simulink model "F16_Without_anti_HWP"  (R2022a)
settings: Solver=ode4  StartTime=0.0  StopTime=200  FixedStep=0.01  RelTol=1e-5  AbsTol=1e-4  EnableMultiTasking=on
InitFcn:
  | F16_Real5_init
libraries: etargetslib x10, dspnetwork x9, simulink x2, vrlib x1
settings Model: SimulationMode=accelerator  Creator=WhisPer  LastModifiedBy=lzj
settings SolverCC: AutoScaleAbsTol=off  AlgebraicLoopSolver=TrustRegion
settings DataIOCC: LimitDataPoints=on  SaveFormat=Array  ReturnWorkspaceOutputs=off
settings OptimizationCC: LifeSpan=inf
settings DebuggingCC: UnderspecifiedInitializationDetection=Classic  MergeDetectMultiDrivingBlocksExec=none  SolverPrmCheckMsg=warning  UnconnectedInputMsg=warning  UnconnectedOutputMsg=warning  UnconnectedLineMsg=warning  StateNameClashWarn=warning  SFUnexpectedBacktrackingDiag=warning  SFNoUnconditionalDefaultTransitionDiag=warning  SFExecutionAtInitializationDiag=none  SFMachineParentedDataDiag=warning  ArithmeticOperatorsInVariantConditions=warning
settings HardwareCC: ProdBitPerPointer=32  ProdBitPerSizeT=32  ProdBitPerPtrDiffT=32  ProdLargestAtomicFloat=None  ProdIntDivRoundTo=Undefined  ProdEndianess=Unspecified  ProdWordSize=32  ProdHWDeviceType=32-bit Generic
settings ModelReferenceCC: PropagateSignalLabelsOutOfModel=off
settings SFSimCC: SimUseLocalCustomCode=off  CustomCodeUndefinedFunction=UseInterfaceOnly
settings RTWCC: RTWUseLocalCustomCode=off
settings CodeAppCC: StateflowObjectComments=on
settings GRTTargetCC: TargetLangStandard=C89/C90 (ANSI)
settings ConfigComp: CovMetricSettings=dw  CovSaveCumulativeToWorkspaceVar=on  CovSaveSingleToWorkspaceVar=on  CovExternalEMLEnable=off

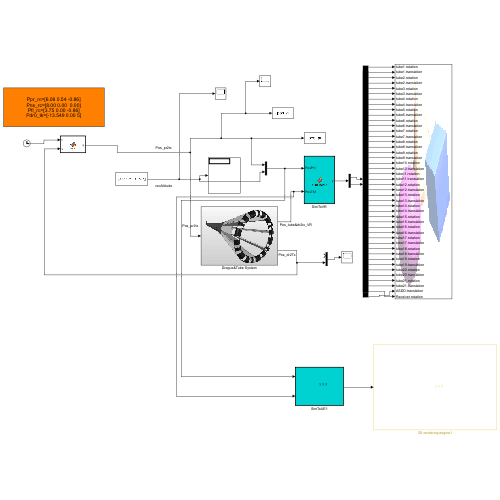
[thumbnail: Simulink's stored preview of the top-level diagram]
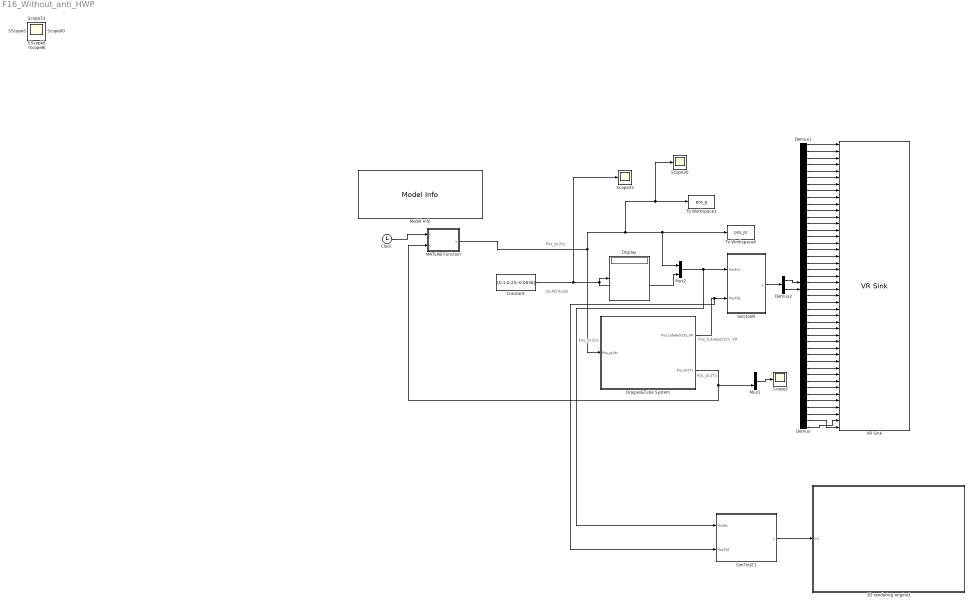
== system F16_Without_anti_HWP ==
  note: recAttitude
  note: Pos_dr2Tx
  note: Pos_tube&dr2tx_VR
  note: Pos_pr2tx
  note: Pos_pr2tx
  3D rendering engine1 : Subsystem
      mask Display: image('C:\Users\lgy13\Desktop\当下要完成的\AirRefueling3DVR-Blank\Icon\sideview.png'); % Use "Edit Image" on toolstrip to change.
  Clock : Clock
  Constant : Constant  Value=[0.1;0.25;-0.0636]
  Demux : Demux  Outputs=22
  Demux1 : Demux  Outputs=22
  Demux2 : Demux  Outputs=[88,66]
  Display : Display
  Drague&Tube System : Subsystem
      mask Display: image(imread('Icon\zhuitao.png'))
  MATLAB Function : MATLAB Function  TreatAsAtomicUnit=on
  Model Info : simulink/Model-Wide Utilities/Model Info  Frame=on  DisplayStringWithTags=|  HorizontalTextAlignment=Center  LeftAlignmentValue=0.5
      | Ppr_rc=[6.06 0.54 -0.86]
      | Pns_rc=[8.00 0.00  0.00]
      | Pfl_rc=[3.75 0.00 -0.86]
      | Pdr0_tk=[-13.549 0.00 5]
  Mux1 : Mux  Inputs=2
  Mux2 : Mux  Inputs=2
  Scope{,1..36} (37 alike) : Scope
  SimToUE1 : MATLAB Function  TreatAsAtomicUnit=on
  SimToVR : MATLAB Function  TreatAsAtomicUnit=on
  To Workspace3 : ToWorkspace  VariableName=pos_g  SampleTime=-1
  To Workspace4 : ToWorkspace  VariableName=pos_pr  SampleTime=-1
  VR Sink : vrlib/VR Sink  InstantiateOnLoad=on  SampleTime=-1  ViewEnable=on  RemoteChange=off  RemoteView=off  FieldsWritten=tube1.rotation.4.1.1.double#tube1.translation.3.1.1.double#tube2.rotation.4.1.1.double#tube2.translation.3.1.1.double#tube3.rotation.4.1.1.double#tube3.translation.3.1.1.double#tube4.rotation.4.1.1.double#tube4.translation.3.1.1.double#tube5.rotation.4.1.1.double#tube5.translation.3.1.1.double#tube6.rotation.4.1.1.double#tube6.translation.3.1.1.double#tube7.rotation.4.1.1.double#tube7.translation.3.1.1.double#tube8.rotation.4.1.1.double#tube8.translation.3.1.1.double#tube9.rotation.4.1.1.double#tube9.translation.3.1.1.double#tube10.rotation.4.1.1.double#tube10.translation.3.1.1.double#tube11.rotation.4.1.1.double#tube11.translation.3.1.1.double#tube12.rotation.4.1.1.double#tube12.translation.3.1.1.double#tube13.rotation.4.1.1.double#tube13.translation.3.1.1.double#tube14.rotation.4.1.1.double#tube14.translation.3.1.1.double#tube15.rotation.4.1.1.double#tube15.translation.3.1.1.double#tube16.rotation.4.1.1.double#tube16.translation.3.1.1.double#tube17.rotation.4.1.1.double#tube17.translation.3.1.1.double#tube18.rotation.4.1.1.double#tube18.translation.3.1.1.double#tube19.rotation.4.1.1.double#tube19.translation.3.1.1.double#tube20.rotation.4.1.1.double#tube20.translation.3.1.1.double#tube21.rotation.4.1.1.double#tube21.translation.3.1.1.double#ASDD.translation.3.1.1.double#Receiver.rotation.4.1.1.double  WorldFileName=AirRefuelingTubeSim.WRL  AutoView=off  VideoDimensions=[]  AllowVariableSize=off
  wires:
  MATLAB Function/1(y) -> Drague&Tube System/1(Pos_pr2tx), Mux2/1, To Workspace4/1, Scope36/1, To Workspace3/1
  Drague&Tube System/2(Pos_dr2Tx) -> MATLAB Function/2(v), Mux1/2
  Mux1/1 -> Scope2/1
  Constant/1 -> Scope35/1, Display/1, Mux2/2
  Demux2/2 -> Demux/1
  SimToVR/1(y) -> Demux2/1
  Drague&Tube System/1(Pos_tube&dr2tx_VR) -> SimToUE1/2(PosTb1), SimToVR/2(PosTb1)
  Mux2/1 -> SimToUE1/1(PosRc), SimToVR/1(PosPr1)
  Demux1/1 -> VR Sink/1
  Demux/1 -> VR Sink/2
  Demux1/2 -> VR Sink/3
  Demux/2 -> VR Sink/4
  Demux1/3 -> VR Sink/5
  Demux/3 -> VR Sink/6
  Demux1/4 -> VR Sink/7
  Demux/4 -> VR Sink/8
  Demux1/5 -> VR Sink/9
  Demux/5 -> VR Sink/10
  Demux1/6 -> VR Sink/11
  Demux/6 -> VR Sink/12
  Demux1/7 -> VR Sink/13
  Demux/7 -> VR Sink/14
  Demux1/8 -> VR Sink/15
  Demux/8 -> VR Sink/16
  Demux1/9 -> VR Sink/17
  Demux/9 -> VR Sink/18
  Demux1/10 -> VR Sink/19
  Demux/10 -> VR Sink/20
  Demux1/11 -> VR Sink/21
  Demux/11 -> VR Sink/22
  Demux1/12 -> VR Sink/23
  Demux/12 -> VR Sink/24
  Demux1/13 -> VR Sink/25
  Demux/13 -> VR Sink/26
  Demux1/14 -> VR Sink/27
  Demux/14 -> VR Sink/28
  Demux1/15 -> VR Sink/29
  Demux/15 -> VR Sink/30
  Demux1/16 -> VR Sink/31
  Demux/16 -> VR Sink/32
  Demux1/17 -> VR Sink/33
  Demux/17 -> VR Sink/34
  Demux1/18 -> VR Sink/35
  Demux/18 -> VR Sink/36
  Demux1/19 -> VR Sink/37
  Demux/19 -> VR Sink/38
  Demux1/20 -> VR Sink/39
  Demux/20 -> VR Sink/40
  Demux1/21 -> VR Sink/41
  Demux/21 -> VR Sink/42
  Demux/22 -> VR Sink/43
  Demux1/22 -> VR Sink/44
  Demux2/1 -> Demux1/1
  Clock/1 -> MATLAB Function/1(t)
  SimToUE1/1(y) -> 3D rendering engine1/1(In1)

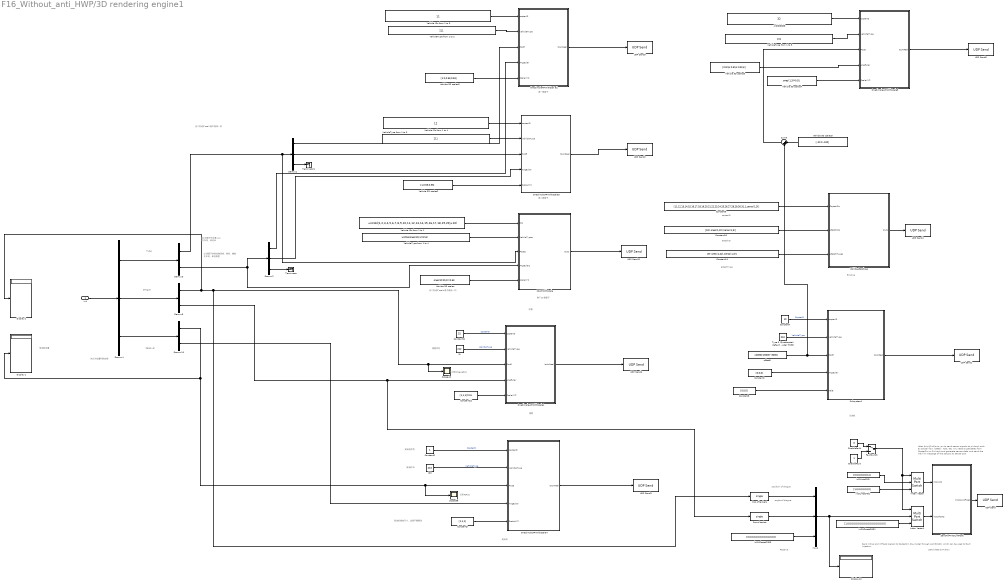
== system F16_Without_anti_HWP/3D rendering engine1 ==
  note: 第一根管子
  note: 这个发送的scale是不是统一的
  note: 受油机位置
  note: 加油机
  note: 锥套
  note: position of drogue
  note: copterID
  note: Send inSILs and inFloats signals to CopterSim DLL model through port 30100, which can be used to fault injection.
  note: 记录RcPos
  note: 20段管子的位置xyz，
      | 北东地，单位米
  note: Note: this API allows you to send sensor signals to pixhawk such as optical flow, battery, ADC, etc. You need to get states from CopterSim or Pixhawk and generate sensor data, and send the mavlink message of the sensors to 30100 port
  note: 锥套序号
  note: attachType
  note: 记录DroguePos
  note: 受油机
  note: Tube
  note: 20段管子的欧拉角滚转、俯仰、偏航
      | 北东地，单位弧度
  note: attachID
  note: 先分为位置和欧拉角
  note: Binding
  note: Send data to Python
  note: Reserve
  note: 软管
  note: 受油机ID
  note: Drogue
  note: angle of drogue
  note: 受油机缩放尺寸，这里不需要改
  note: Receiver
  note: 受油机序号
  note: 这个发送的scale是不是统一的
  note: 第二根管子
  note: 剩下18根管子
  In1 : Inport
  20APIWithScale : Subsystem
  Constant1 : Constant  Value=[0,0,0]
  Constant10 : Constant  Value=[10* ones(1,22),zeros(1,3)]
  Constant11 : Constant  Value=[3* ones(1,22),zeros(1,3)]
  Constant2 : Constant
  Constant21 : Constant  Value=31
  Constant22 : Constant  Value=[1,1,1]*0.5
  Constant3 : Constant  Value=[1,1,1]
  Constant7 : Constant  Value=10
  Constant8 : Constant  Value=[0,0,0]
  Constant9 : Constant  Value=[11,12,13,14,15,16,17,18,19,20,21,22,23,24,25,26,27,28,29,30,31,1,zeros(1,3)]
  Demux1 : Demux  Outputs=[3,3,54]
  Demux10 : Demux  Outputs=[3,3]
  Demux2 : Demux  Outputs=[3,3,54]
  Demux3 : Demux  Outputs=[60,60]
  Demux4 : Demux  Outputs=[120,6,6]
  Demux5 : Demux  Outputs=[3,3]
  DisableFault : Constant  Value=0
  Display1 : Display
  Display10 : Display
  Display2 : Display
  EnableFault : Constant
  FaultSwitch : ManualSwitch
  ID : Constant  Value=212
  ID3 : Constant  Value=213
  Index Vector : MultiPortSwitch  DataPortOrder=Zero-based contiguous  Inputs=2  zeroidx=on  SaturateOnIntegerOverflow=off  InputSameDT=off
  Index Vector1 : MultiPortSwitch  DataPortOrder=Zero-based contiguous  Inputs=2  zeroidx=on  SaturateOnIntegerOverflow=off  InputSameDT=off
  Mux2 : Mux  Inputs=[3 3 14]
  OneSimpleAPIWithScal e2 : Subsystem
  OneSimpleAPIWithScale1 : Subsystem
  OneSimpleAPIWithScale3 : Subsystem
  OneSimpleAPIWithScale4 : Subsystem
  OneSimpleAPIWithScale5 : Subsystem
  Pos of tanker : DataTypeConversion  OutDataTypeStr=single  SaturateOnIntegerOverflow=off  RndMeth=Floor
  Pos of tanker1 : DataTypeConversion  OutDataTypeStr=single  SaturateOnIntegerOverflow=off  RndMeth=Floor
  Scope38 : Scope
  Scope40 : Scope
  SendToPX4SILIntFloat : Subsystem
  Subsystem1 : Subsystem
  Sum5 : Sum  Inputs=|++
  Terminator : Terminator
  Terminator1 : Terminator
  "Type 3 (Quadcopter), default model (F450)" : Constant  Value=210
  UDP Send : dspnetwork/UDP Send  remoteURL='224.0.0.10'  remotePort=20006  localURL='0.0.0.0'  localPortSource=Automatically determine  localPort=-1  sendBufferSize=8192  sampletime=-1  blockPlatform=[]  separateLengthPort=0
  UDP Send{1..6,8,11} (8 alike) : dspnetwork/UDP Send  remoteURL='127.0.0.1'  remotePort=20010  localURL='0.0.0.0'  localPortSource=Automatically determine  localPort=-1  sendBufferSize=8192  sampletime=-1  blockPlatform=[]  separateLengthPort=0
  Vehicle 3D scales : Constant  Value=ones(3*20,1)*0.53
  Vehicle 3D scales2 : Constant  Value=[1,0.53,0.53]
  Vehicle 3D scales3 : Constant  Value=[1.2,0.53,0.53]
  Vehicle 3D scales4 : Constant  Value=ones(1,3)*0.01
  Vehicle 3D scales5 : Constant  Value=[-20 0 -100]
  Vehicle 3D scales6 : Constant  Value=[0.5*pi 0.5*pi 0.5*pi]
  Vehicle IDs from 1 to 1 : Constant  Value=uint16([1,2,3,4,5,6,7,8,9,10,11,12,13,14,15,16,17,18,19,20]+10)
  Vehicle IDs from 1 to 3 : Constant  Value=11
  Vehicle IDs from 1 to 4 : Constant  Value=12
  VehicleAttatchreq : Subsystem
  VehicleType from 1 to 2 : Constant  Value=211
  VehicleType from 1 to 3 : Constant  Value=211
  VehicleType from 1 to 4 : Constant  Value=uint16(ones(20,1)*211)
  VehicleType from 1 to 5 : Constant  Value=211
  inSILFloatsCMD1 : Constant  Value=[1,0,0,0,0,0,0,0,0,0,0,0,0,0,0,0,0,0,0,0]  OutDataTypeStr=single
  inSILFloatsCMD3 : Constant  Value=[0,0,0,0,0,0,0,0,0,0,0,0,0,0]  OutDataTypeStr=single
  inSILIntsCMD : Constant  Value=[0,0,0,0,0,0,0,1]  OutDataTypeStr=int32
  inSILIntsCMD1 : Constant  Value=[1,0,0,0,0,0,0,0]  OutDataTypeStr=int32
  offset5 : Constant  Value=[20000 20000 -3000]
  上帝视角观察 : Constant  Value=32
  wires:
  inSILFloatsCMD3/1 -> Mux2/3
  Demux5/1 -> Display2/1, Pos of tanker1/1, Scope40/1, OneSimpleAPIWithScale1/3(PosE)
  Mux2/1 -> Display10/1, Index Vector1/2
  Constant11/1 -> VehicleAttatchreq/3(AttatchTypes)
  Constant1/1 -> Subsystem1/4(AngEuler)
  Constant10/1 -> VehicleAttatchreq/2(AttatchIDs)
  Constant9/1 -> VehicleAttatchreq/1(CopterIDs)
  DisableFault/1 -> FaultSwitch/1
  "Type 3 (Quadcopter), default model (F450)"/1 -> Subsystem1/2(vehicleType)  "VehicleType"
  In1/1 -> Demux4/1
  Constant21/1 -> OneSimpleAPIWithScale1/1(copterID)  "CopterID"
  OneSimpleAPIWithScale4/1(toUnReal) -> UDP Send3/1
  Pos of tanker1/1 -> Mux2/1
  Constant8/1 -> Subsystem1/5(VelE)
  20APIWithScale/1(Out1) -> UDP Send11/1
  Constant2/1 -> OneSimpleAPIWithScale4/1(copterID)  "CopterID"
  OneSimpleAPIWithScale1/1(toUnReal) -> UDP Send6/1
  Constant22/1 -> OneSimpleAPIWithScale1/5(ScaleXYZ)
  inSILIntsCMD/1 -> Index Vector/2
  Vehicle IDs from 1 to 1/1 -> 20APIWithScale/1(IDs)
  inSILIntsCMD1/1 -> Index Vector/3
  Constant3/1 -> OneSimpleAPIWithScale4/5(ScaleXYZ)
  Demux4/1 -> Demux3/1
  Constant7/1 -> Subsystem1/1(copterID)  "CopterID"
  FaultSwitch/1 -> Index Vector1/1, Index Vector/1
  Demux5/2 -> Pos of tanker/1, OneSimpleAPIWithScale1/4(AngEuler)
  Index Vector/1 -> SendToPX4SILIntFloat/1(inSILInts)
  ID/1 -> OneSimpleAPIWithScale1/2(vehicleType)  "VehicleType"
  Index Vector1/1 -> SendToPX4SILIntFloat/2(inSILFloats)
  Demux4/3 -> Demux10/1
  SendToPX4SILIntFloat/1(PX4SILIntFloat) -> UDP Send/1
  Demux10/2 -> OneSimpleAPIWithScale4/4(AngEuler)
  Subsystem1/1(toUnReal) -> UDP Send1/1
  ID3/1 -> OneSimpleAPIWithScale4/2(vehicleType)  "VehicleType"
  Pos of tanker/1 -> Mux2/2
  EnableFault/1 -> FaultSwitch/2
  inSILFloatsCMD1/1 -> Index Vector1/3
  VehicleType from 1 to 4/1 -> 20APIWithScale/2(VehileTypes)
  VehicleAttatchreq/1(Out1) -> UDP Send4/1
  Demux4/2 -> Demux5/1
  Demux3/1 -> Demux1/1, 20APIWithScale/3(PosEs)
  Vehicle 3D scales/1 -> 20APIWithScale/5(scaleXYZ)
  OneSimpleAPIWithScale3/1(toUnReal) -> UDP Send2/1
  OneSimpleAPIWithScal e2/1(toUnReal) -> UDP Send5/1
  Vehicle IDs from 1 to 3/1 -> OneSimpleAPIWithScal e2/1(copterID)
  VehicleType from 1 to 2/1 -> OneSimpleAPIWithScal e2/2(vehicleType)
  Vehicle IDs from 1 to 4/1 -> OneSimpleAPIWithScale3/1(copterID)
  VehicleType from 1 to 3/1 -> OneSimpleAPIWithScale3/2(vehicleType)
  Vehicle 3D scales3/1 -> OneSimpleAPIWithScal e2/5(ScaleXYZ)
  Vehicle 3D scales2/1 -> OneSimpleAPIWithScale3/5(ScaleXYZ)
  Demux1/1 -> OneSimpleAPIWithScal e2/3(PosE)
  Demux1/2 -> OneSimpleAPIWithScale3/3(PosE)
  Demux2/1 -> OneSimpleAPIWithScal e2/4(AngEuler)
  Demux2/2 -> OneSimpleAPIWithScale3/4(AngEuler)
  Demux3/2 -> Demux2/1, 20APIWithScale/4(AngEulers)
  Demux2/3 -> Terminator/1
  Demux1/3 -> Terminator1/1
  Demux10/1 -> Scope38/1, OneSimpleAPIWithScale4/3(PosE), Display1/1
  OneSimpleAPIWithScale5/1(toUnReal) -> UDP Send8/1
  上帝视角观察/1 -> OneSimpleAPIWithScale5/1(copterID)
  Vehicle 3D scales4/1 -> OneSimpleAPIWithScale5/5(ScaleXYZ)
  VehicleType from 1 to 5/1 -> OneSimpleAPIWithScale5/2(vehicleType)
  Vehicle 3D scales6/1 -> OneSimpleAPIWithScale5/4(AngEuler)
  offset5/1 -> Sum5/2, Subsystem1/3(PosE)
  Vehicle 3D scales5/1 -> Sum5/1
  Sum5/1 -> OneSimpleAPIWithScale5/3(PosE)

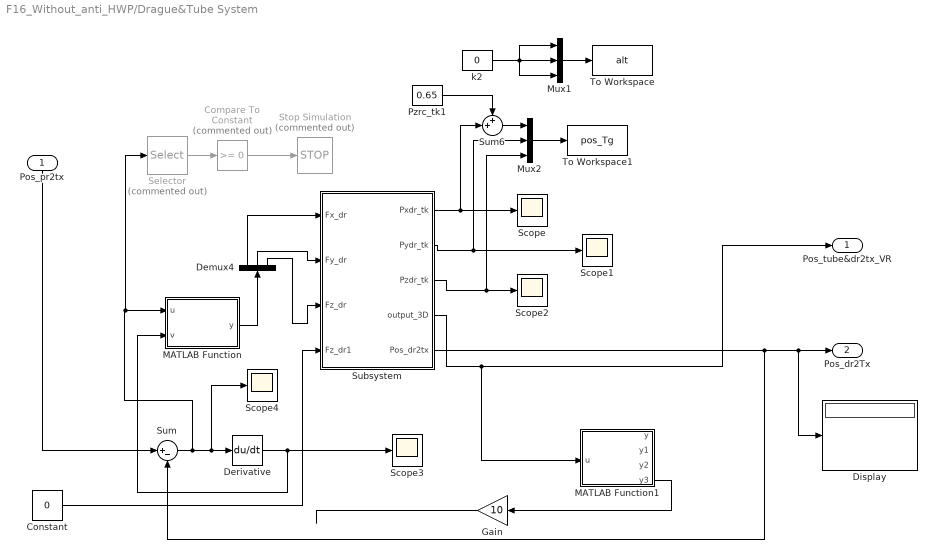
== system F16_Without_anti_HWP/Drague&Tube System ==
  Pos_pr2tx : Inport
  Compare To Constant : simulink/Logic and Bit Operations/Compare To Constant  Commented=on  relop=>=  const=0  OutDataTypeStr=boolean
  Constant : Constant  Value=0
  Demux4 : Demux  Outputs=3
  Derivative : Derivative
  Display : Display
  Gain : Gain  Gain=10
  MATLAB Function : MATLAB Function  TreatAsAtomicUnit=on
  MATLAB Function1 : MATLAB Function  TreatAsAtomicUnit=on
  Mux1 : Mux  Inputs=3
  Mux2 : Mux  Inputs=3
  Pzrc_tk1 : Constant  Value=0.65
  Scope{,1..4} (5 alike) : Scope
  Selector : Selector  Commented=on  InputPortWidth=3  IndexOptions=Index vector (dialog)  Indices=[1]  OutputSizes=1
  Stop Simulation : Stop  Commented=on
  Subsystem : Subsystem
  Sum : Sum  Inputs=|+-
  Sum6 : Sum  Inputs=++|
  To Workspace : ToWorkspace  VariableName=alt  SampleTime=-1
  To Workspace1 : ToWorkspace  VariableName=pos_Tg  SampleTime=-1
  k2 : Constant  Value=0
  Pos_tube&dr2tx_VR : Outport
  Pos_dr2Tx : Outport  Port=2
  wires:
  Subsystem/5(Pos_dr2tx) -> Sum/2, Display/1, Pos_dr2Tx/1
  Subsystem/3(Pzdr_tk) -> Mux2/3, Scope2/1
  Subsystem/1(Pxdr_tk) -> Scope/1, Sum6/2
  Subsystem/2(Pydr_tk) -> Mux2/2, Scope1/1
  Mux2/1 -> To Workspace1/1
  Mux1/1 -> To Workspace/1
  Pzrc_tk1/1 -> Sum6/1
  k2/1 -> Mux1/3, Mux1/1, Mux1/2
  Sum6/1 -> Mux2/1
  Subsystem/4(output_3D) -> MATLAB Function1/1(u), Pos_tube&dr2tx_VR/1
  Demux4/1 -> Subsystem/1(Fx_dr)
  Demux4/2 -> Subsystem/2(Fy_dr)
  Demux4/3 -> Subsystem/3(Fz_dr)
  Pos_pr2tx/1 -> Sum/1
  Sum/1 -> Selector/1, MATLAB Function/1(u), Scope4/1, Derivative/1
  Derivative/1 -> MATLAB Function/2(v), Scope3/1
  MATLAB Function/1(y) -> Demux4/1
  Compare To Constant/1 -> Stop Simulation/1
  Selector/1 -> Compare To Constant/1
  MATLAB Function1/4(y3) -> Gain/1
  Gain/1 -> ?
  Constant/1 -> Subsystem/4(Fz_dr1)

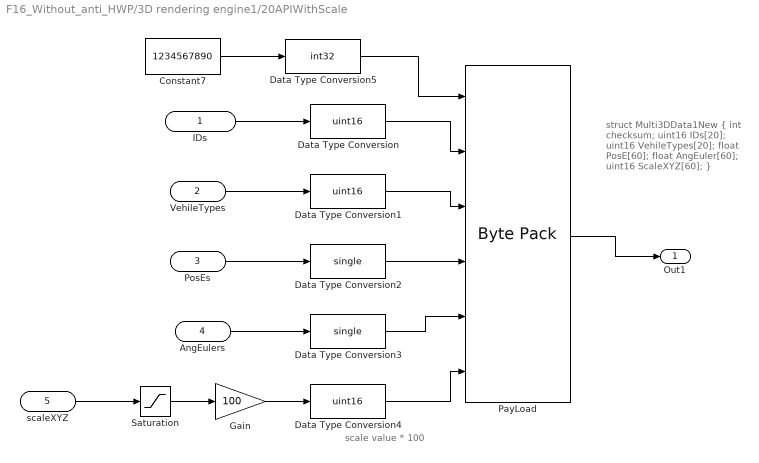
== system F16_Without_anti_HWP/3D rendering engine1/20APIWithScale ==
  note: struct Multi3DData1New {
      |        int checksum;
      | 	uint16 IDs[20];
      | 	uint16 VehileTypes[20];
      | 	float PosE[60];
      | 	float AngEuler[60];
      | 	uint16 ScaleXYZ[60];
      | }
  note: scale value * 100
  IDs : Inport  PortDimensions=20
  VehileTypes : Inport  Port=2  PortDimensions=20
  PosEs : Inport  Port=3  PortDimensions=60
  AngEulers : Inport  Port=4  PortDimensions=60
  scaleXYZ : Inport  Port=5  PortDimensions=60
  Constant7 : Constant  Value=1234567890
  Data Type Conversion : DataTypeConversion  OutDataTypeStr=uint16  SaturateOnIntegerOverflow=off  RndMeth=Floor
  Data Type Conversion1 : DataTypeConversion  OutDataTypeStr=uint16  SaturateOnIntegerOverflow=off  RndMeth=Floor
  Data Type Conversion2 : DataTypeConversion  OutDataTypeStr=single  SaturateOnIntegerOverflow=off  RndMeth=Floor
  Data Type Conversion3 : DataTypeConversion  OutDataTypeStr=single  SaturateOnIntegerOverflow=off  RndMeth=Floor
  Data Type Conversion4 : DataTypeConversion  OutDataTypeStr=uint16  SaturateOnIntegerOverflow=off  RndMeth=Floor
  Data Type Conversion5 : DataTypeConversion  OutDataTypeStr=int32  SaturateOnIntegerOverflow=off  RndMeth=Floor
  Gain : Gain  Gain=100
  PayLoad : etargetslib/Byte Pack  datatypes={'int32','uint16','uint16','single','single','uint16'}  byteAlign=4
  Saturation : Saturate  UpperLimit=655.35  LowerLimit=0.01
  Out1 : Outport  VectorParamsAs1DForOutWhenUnconnected=off
  wires:
  Data Type Conversion3/1 -> PayLoad/5
  Data Type Conversion1/1 -> PayLoad/3
  PosEs/1 -> Data Type Conversion2/1
  Data Type Conversion2/1 -> PayLoad/4
  AngEulers/1 -> Data Type Conversion3/1
  PayLoad/1 -> Out1/1
  VehileTypes/1 -> Data Type Conversion1/1
  Data Type Conversion/1 -> PayLoad/2
  IDs/1 -> Data Type Conversion/1
  scaleXYZ/1 -> Saturation/1
  Data Type Conversion4/1 -> PayLoad/6
  Saturation/1 -> Gain/1
  Gain/1 -> Data Type Conversion4/1
  Constant7/1 -> Data Type Conversion5/1
  Data Type Conversion5/1 -> PayLoad/1

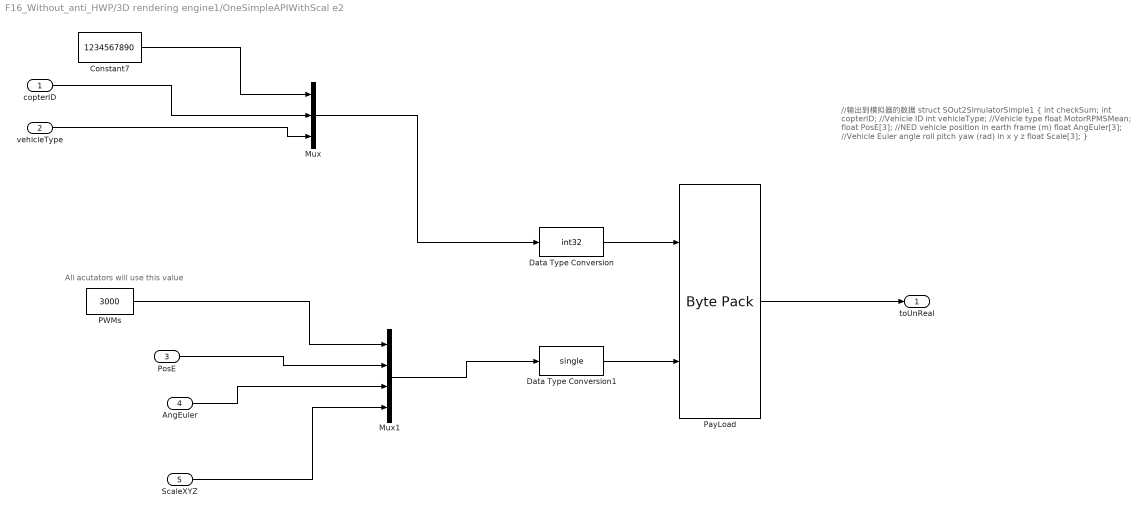
== system F16_Without_anti_HWP/3D rendering engine1/OneSimpleAPIWithScal e2 ==
  note: //输出到模拟器的数据
      | struct SOut2SimulatorSimple1 {
      | 	int checkSum;
      | 	int copterID;  //Vehicle ID
      | 	int vehicleType;  //Vehicle type
      | 	float MotorRPMSMean;
      | 	float PosE[3];   //NED vehicle position in earth frame (m)
      | 	float AngEuler[3];  //Vehicle Euler angle roll pitch yaw (rad) in x y z
      | 	float Scale[3];
      | }
  note: All acutators will use this value
  copterID : Inport  PortDimensions=1
  vehicleType : Inport  Port=2  PortDimensions=1
  PosE : Inport  Port=3  PortDimensions=3
  AngEuler : Inport  Port=4  PortDimensions=3
  ScaleXYZ : Inport  Port=5  PortDimensions=3
  Constant7 : Constant  Value=1234567890
  Data Type Conversion : DataTypeConversion  OutDataTypeStr=int32  SaturateOnIntegerOverflow=off  RndMeth=Floor
  Data Type Conversion1 : DataTypeConversion  OutDataTypeStr=single  SaturateOnIntegerOverflow=off  RndMeth=Floor
  Mux : Mux  Inputs=3
  Mux1 : Mux
  PWMs : Constant  Value=3000
  PayLoad : etargetslib/Byte Pack  datatypes={'int32','single'}  byteAlign=1
  toUnReal : Outport  VectorParamsAs1DForOutWhenUnconnected=off
  wires:
  PayLoad/1 -> toUnReal/1
  Data Type Conversion/1 -> PayLoad/1
  Data Type Conversion1/1 -> PayLoad/2
  copterID/1 -> Mux/2
  vehicleType/1 -> Mux/3
  Constant7/1 -> Mux/1
  Mux/1 -> Data Type Conversion/1
  Mux1/1 -> Data Type Conversion1/1
  PWMs/1 -> Mux1/1
  PosE/1 -> Mux1/2
  AngEuler/1 -> Mux1/3
  ScaleXYZ/1 -> Mux1/4

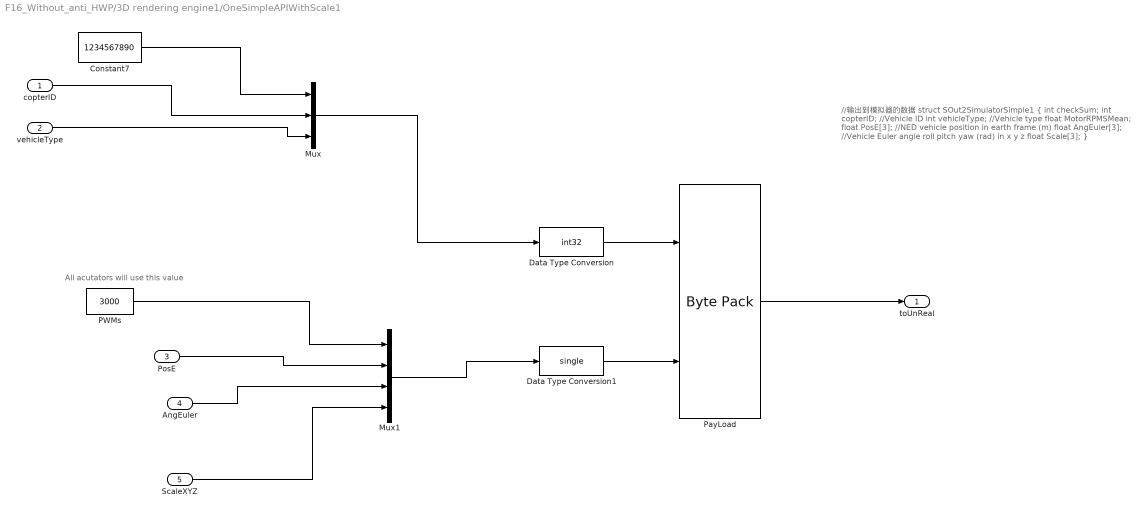
== system F16_Without_anti_HWP/3D rendering engine1/OneSimpleAPIWithScale1 ==
  note: //输出到模拟器的数据
      | struct SOut2SimulatorSimple1 {
      | 	int checkSum;
      | 	int copterID;  //Vehicle ID
      | 	int vehicleType;  //Vehicle type
      | 	float MotorRPMSMean;
      | 	float PosE[3];   //NED vehicle position in earth frame (m)
      | 	float AngEuler[3];  //Vehicle Euler angle roll pitch yaw (rad) in x y z
      | 	float Scale[3];
      | }
  note: All acutators will use this value
  copterID : Inport  PortDimensions=1
  vehicleType : Inport  Port=2  PortDimensions=1
  PosE : Inport  Port=3  PortDimensions=3
  AngEuler : Inport  Port=4  PortDimensions=3
  ScaleXYZ : Inport  Port=5  PortDimensions=3
  Constant7 : Constant  Value=1234567890
  Data Type Conversion : DataTypeConversion  OutDataTypeStr=int32  SaturateOnIntegerOverflow=off  RndMeth=Floor
  Data Type Conversion1 : DataTypeConversion  OutDataTypeStr=single  SaturateOnIntegerOverflow=off  RndMeth=Floor
  Mux : Mux  Inputs=3
  Mux1 : Mux
  PWMs : Constant  Value=3000
  PayLoad : etargetslib/Byte Pack  datatypes={'int32','single'}  byteAlign=1
  toUnReal : Outport  VectorParamsAs1DForOutWhenUnconnected=off
  wires:
  PayLoad/1 -> toUnReal/1
  Data Type Conversion/1 -> PayLoad/1
  Data Type Conversion1/1 -> PayLoad/2
  copterID/1 -> Mux/2
  vehicleType/1 -> Mux/3
  Constant7/1 -> Mux/1
  Mux/1 -> Data Type Conversion/1
  Mux1/1 -> Data Type Conversion1/1
  PWMs/1 -> Mux1/1
  PosE/1 -> Mux1/2
  AngEuler/1 -> Mux1/3
  ScaleXYZ/1 -> Mux1/4

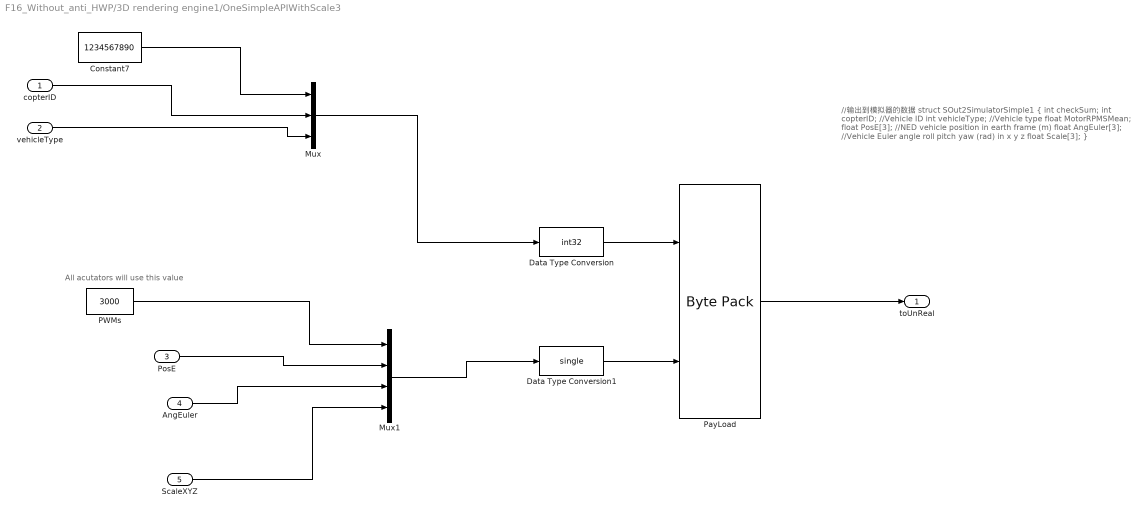
== system F16_Without_anti_HWP/3D rendering engine1/OneSimpleAPIWithScale3 ==
  note: All acutators will use this value
  note: //输出到模拟器的数据
      | struct SOut2SimulatorSimple1 {
      | 	int checkSum;
      | 	int copterID;  //Vehicle ID
      | 	int vehicleType;  //Vehicle type
      | 	float MotorRPMSMean;
      | 	float PosE[3];   //NED vehicle position in earth frame (m)
      | 	float AngEuler[3];  //Vehicle Euler angle roll pitch yaw (rad) in x y z
      | 	float Scale[3];
      | }
  copterID : Inport  PortDimensions=1
  vehicleType : Inport  Port=2  PortDimensions=1
  PosE : Inport  Port=3  PortDimensions=3
  AngEuler : Inport  Port=4  PortDimensions=3
  ScaleXYZ : Inport  Port=5  PortDimensions=3
  Constant7 : Constant  Value=1234567890
  Data Type Conversion : DataTypeConversion  OutDataTypeStr=int32  SaturateOnIntegerOverflow=off  RndMeth=Floor
  Data Type Conversion1 : DataTypeConversion  OutDataTypeStr=single  SaturateOnIntegerOverflow=off  RndMeth=Floor
  Mux : Mux  Inputs=3
  Mux1 : Mux
  PWMs : Constant  Value=3000
  PayLoad : etargetslib/Byte Pack  datatypes={'int32','single'}  byteAlign=1
  toUnReal : Outport  VectorParamsAs1DForOutWhenUnconnected=off
  wires:
  ScaleXYZ/1 -> Mux1/4
  AngEuler/1 -> Mux1/3
  PosE/1 -> Mux1/2
  PWMs/1 -> Mux1/1
  Mux1/1 -> Data Type Conversion1/1
  Mux/1 -> Data Type Conversion/1
  Constant7/1 -> Mux/1
  vehicleType/1 -> Mux/3
  copterID/1 -> Mux/2
  Data Type Conversion1/1 -> PayLoad/2
  Data Type Conversion/1 -> PayLoad/1
  PayLoad/1 -> toUnReal/1

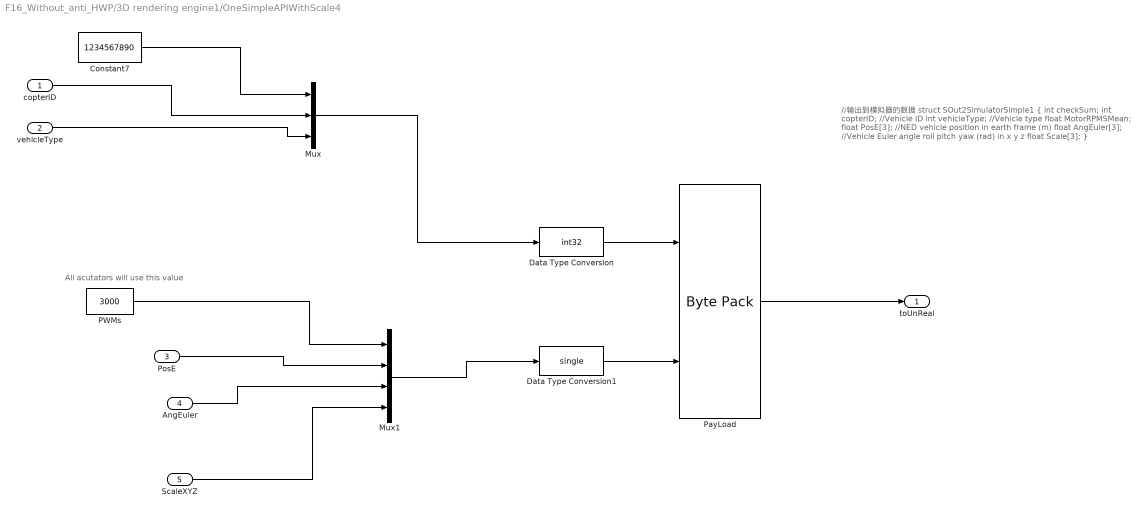
== system F16_Without_anti_HWP/3D rendering engine1/OneSimpleAPIWithScale4 ==
  note: All acutators will use this value
  note: //输出到模拟器的数据
      | struct SOut2SimulatorSimple1 {
      | 	int checkSum;
      | 	int copterID;  //Vehicle ID
      | 	int vehicleType;  //Vehicle type
      | 	float MotorRPMSMean;
      | 	float PosE[3];   //NED vehicle position in earth frame (m)
      | 	float AngEuler[3];  //Vehicle Euler angle roll pitch yaw (rad) in x y z
      | 	float Scale[3];
      | }
  copterID : Inport  PortDimensions=1
  vehicleType : Inport  Port=2  PortDimensions=1
  PosE : Inport  Port=3  PortDimensions=3
  AngEuler : Inport  Port=4  PortDimensions=3
  ScaleXYZ : Inport  Port=5  PortDimensions=3
  Constant7 : Constant  Value=1234567890
  Data Type Conversion : DataTypeConversion  OutDataTypeStr=int32  SaturateOnIntegerOverflow=off  RndMeth=Floor
  Data Type Conversion1 : DataTypeConversion  OutDataTypeStr=single  SaturateOnIntegerOverflow=off  RndMeth=Floor
  Mux : Mux  Inputs=3
  Mux1 : Mux
  PWMs : Constant  Value=3000
  PayLoad : etargetslib/Byte Pack  datatypes={'int32','single'}  byteAlign=1
  toUnReal : Outport  VectorParamsAs1DForOutWhenUnconnected=off
  wires:
  ScaleXYZ/1 -> Mux1/4
  AngEuler/1 -> Mux1/3
  PosE/1 -> Mux1/2
  PWMs/1 -> Mux1/1
  Mux1/1 -> Data Type Conversion1/1
  Mux/1 -> Data Type Conversion/1
  Constant7/1 -> Mux/1
  vehicleType/1 -> Mux/3
  copterID/1 -> Mux/2
  Data Type Conversion1/1 -> PayLoad/2
  Data Type Conversion/1 -> PayLoad/1
  PayLoad/1 -> toUnReal/1

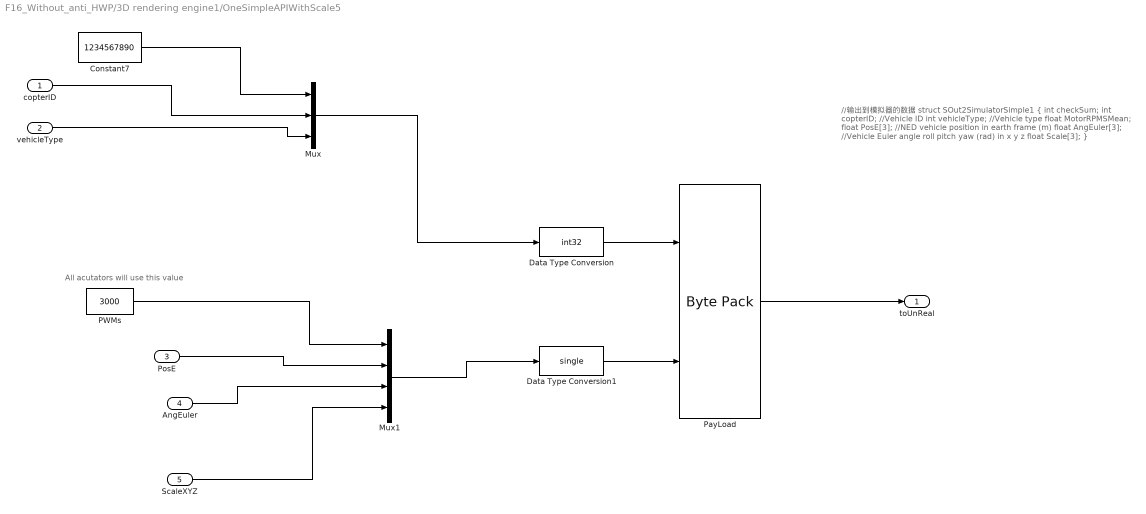
== system F16_Without_anti_HWP/3D rendering engine1/OneSimpleAPIWithScale5 ==
  note: //输出到模拟器的数据
      | struct SOut2SimulatorSimple1 {
      | 	int checkSum;
      | 	int copterID;  //Vehicle ID
      | 	int vehicleType;  //Vehicle type
      | 	float MotorRPMSMean;
      | 	float PosE[3];   //NED vehicle position in earth frame (m)
      | 	float AngEuler[3];  //Vehicle Euler angle roll pitch yaw (rad) in x y z
      | 	float Scale[3];
      | }
  note: All acutators will use this value
  copterID : Inport  PortDimensions=1
  vehicleType : Inport  Port=2  PortDimensions=1
  PosE : Inport  Port=3  PortDimensions=3
  AngEuler : Inport  Port=4  PortDimensions=3
  ScaleXYZ : Inport  Port=5  PortDimensions=3
  Constant7 : Constant  Value=1234567890
  Data Type Conversion : DataTypeConversion  OutDataTypeStr=int32  SaturateOnIntegerOverflow=off  RndMeth=Floor
  Data Type Conversion1 : DataTypeConversion  OutDataTypeStr=single  SaturateOnIntegerOverflow=off  RndMeth=Floor
  Mux : Mux  Inputs=3
  Mux1 : Mux
  PWMs : Constant  Value=3000
  PayLoad : etargetslib/Byte Pack  datatypes={'int32','single'}  byteAlign=1
  toUnReal : Outport  VectorParamsAs1DForOutWhenUnconnected=off
  wires:
  PayLoad/1 -> toUnReal/1
  Data Type Conversion/1 -> PayLoad/1
  Data Type Conversion1/1 -> PayLoad/2
  copterID/1 -> Mux/2
  vehicleType/1 -> Mux/3
  Constant7/1 -> Mux/1
  Mux/1 -> Data Type Conversion/1
  Mux1/1 -> Data Type Conversion1/1
  PWMs/1 -> Mux1/1
  PosE/1 -> Mux1/2
  AngEuler/1 -> Mux1/3
  ScaleXYZ/1 -> Mux1/4

== system F16_Without_anti_HWP/3D rendering engine1/SendToPX4SILIntFloat ==
  note: struct PX4SILIntFloat {
      | int checksum ;
      | int CopterID ;
      | int inSILInts [ 8 ];
      | float inSILFLoats [ 20 ];
      | }
  note: This message will be sent to PX4 DLL model's input signals inSILInts[8] and inSILFloats[20].
      | The checksum should be set to 1234567897, and the data should be sent to port 30100+(i-1)*2
  inSILInts : Inport  OutDataTypeStr=int32  PortDimensions=8
  inSILFloats : Inport  Port=2  OutDataTypeStr=single  PortDimensions=20
  CopterID : Constant  Value=10  OutDataTypeStr=Inherit: Inherit via back propagation
  Data Type Conversion1 : DataTypeConversion  OutDataTypeStr=int32  SaturateOnIntegerOverflow=off  RndMeth=Floor
  Data Type Conversion2 : DataTypeConversion  OutDataTypeStr=single  SaturateOnIntegerOverflow=off  RndMeth=Floor
  Data Type Conversion3 : DataTypeConversion  OutDataTypeStr=int32  SaturateOnIntegerOverflow=off  RndMeth=Floor
  Mux : Mux  Inputs=2
  PayLoad : etargetslib/Byte Pack  datatypes={'int32','int32','single'}  byteAlign=8
  checksum : Constant  Value=1234567897  OutDataTypeStr=Inherit: Inherit via back propagation
  PX4SILIntFloat : Outport  OutDataTypeStr=uint8  PortDimensions=120  VectorParamsAs1DForOutWhenUnconnected=off
  wires:
  inSILFloats/1 -> Data Type Conversion2/1
  inSILInts/1 -> Data Type Conversion1/1
  PayLoad/1 -> PX4SILIntFloat/1
  Data Type Conversion1/1 -> PayLoad/2
  Data Type Conversion2/1 -> PayLoad/3
  checksum/1 -> Mux/1
  Mux/1 -> Data Type Conversion3/1
  Data Type Conversion3/1 -> PayLoad/1
  CopterID/1 -> Mux/2

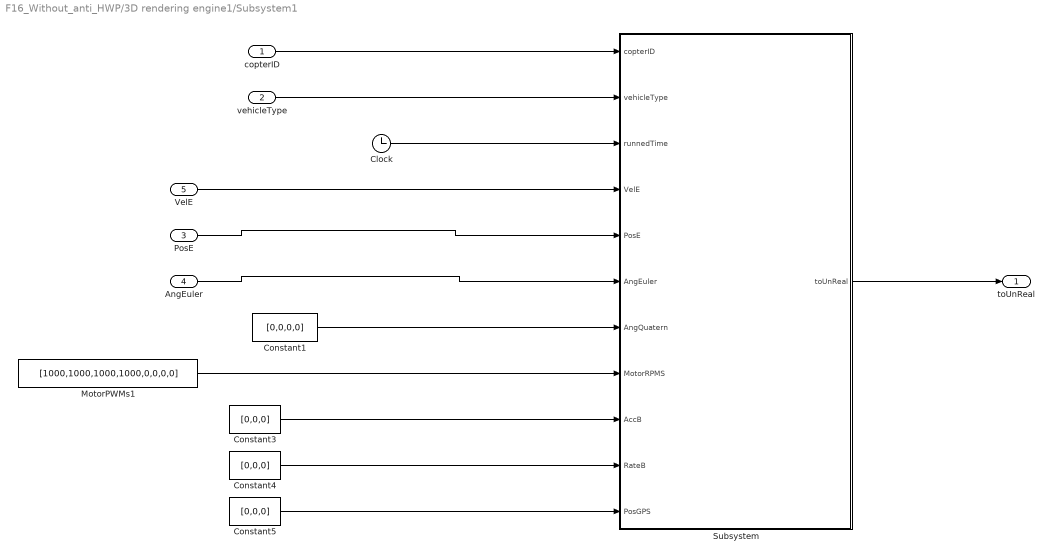
== system F16_Without_anti_HWP/3D rendering engine1/Subsystem1 ==
  copterID : Inport  PortDimensions=1
  vehicleType : Inport  Port=2  PortDimensions=1
  PosE : Inport  Port=3  PortDimensions=3
  AngEuler : Inport  Port=4  PortDimensions=3
  VelE : Inport  Port=5  PortDimensions=3
  Clock : Clock
  Constant1 : Constant  Value=[0,0,0,0]
  Constant3 : Constant  Value=[0,0,0]
  Constant4 : Constant  Value=[0,0,0]
  Constant5 : Constant  Value=[0,0,0]
  MotorPWMs1 : Constant  Value=[1000,1000,1000,1000,0,0,0,0]
  Subsystem : Subsystem
  toUnReal : Outport  VectorParamsAs1DForOutWhenUnconnected=off
  wires:
  VelE/1 -> Subsystem/4("VelE ")
  PosE/1 -> Subsystem/5(PosE)
  vehicleType/1 -> Subsystem/2(vehicleType)
  Clock/1 -> Subsystem/3(runnedTime)
  Constant4/1 -> Subsystem/10(RateB)
  Constant5/1 -> Subsystem/11(PosGPS)
  AngEuler/1 -> Subsystem/6(AngEuler)
  Subsystem/1(toUnReal) -> toUnReal/1
  Constant3/1 -> Subsystem/9(AccB)
  Constant1/1 -> Subsystem/7(AngQuatern)
  copterID/1 -> Subsystem/1(copterID)
  MotorPWMs1/1 -> Subsystem/8(MotorRPMS)

== system F16_Without_anti_HWP/3D rendering engine1/VehicleAttatchreq ==
  note: struct VehicleAttatch25 {
      | 	int checksum;//1234567892
      | 	int CopterIDs[25];
      | 	int AttatchIDs[25];
      | 	int AttatchTypes[25];//0：正常模式，1：相对位置不相对姿态，2：相对位置+偏航（不相对俯仰和滚转），3：相对位置+全姿态（俯仰滚转偏航）
      | }
  CopterIDs : Inport  PortDimensions=25
  AttatchIDs : Inport  Port=2  PortDimensions=25
  AttatchTypes : Inport  Port=3  PortDimensions=25
  Constant7 : Constant  Value=1234567892
  Data Type Conversion{,1..2,4} (4 alike) : DataTypeConversion  OutDataTypeStr=int32  SaturateOnIntegerOverflow=off  RndMeth=Floor
  PayLoad : etargetslib/Byte Pack  datatypes={'int32','int32','int32','int32'}  byteAlign=4
  Out1 : Outport  VectorParamsAs1DForOutWhenUnconnected=off
  wires:
  Data Type Conversion1/1 -> PayLoad/3
  AttatchTypes/1 -> Data Type Conversion2/1
  Data Type Conversion2/1 -> PayLoad/4
  PayLoad/1 -> Out1/1
  AttatchIDs/1 -> Data Type Conversion1/1
  Data Type Conversion/1 -> PayLoad/2
  CopterIDs/1 -> Data Type Conversion/1
  Constant7/1 -> Data Type Conversion4/1
  Data Type Conversion4/1 -> PayLoad/1

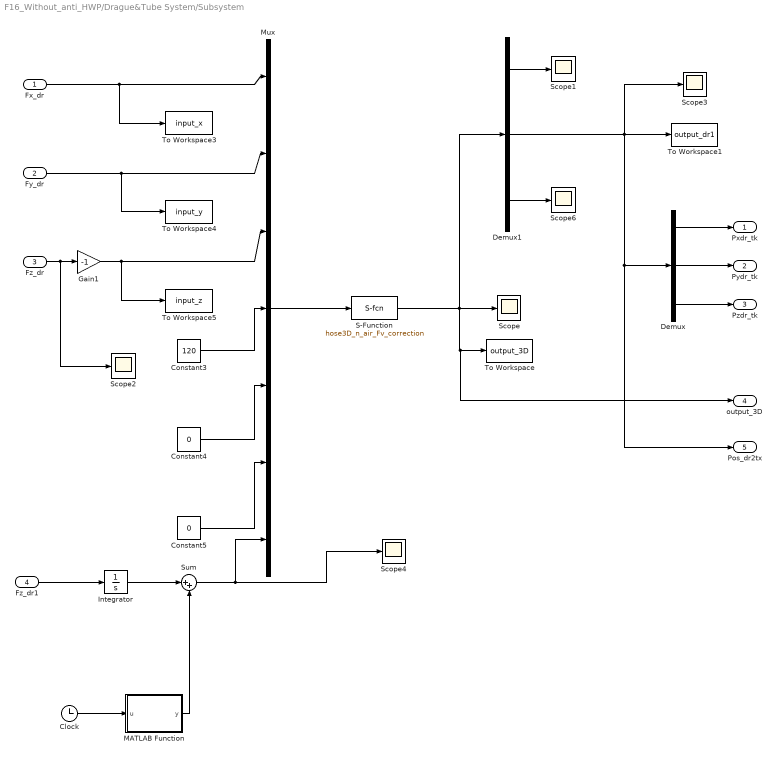
== system F16_Without_anti_HWP/Drague&Tube System/Subsystem ==
  Fx_dr : Inport
  Fy_dr : Inport  Port=2
  Fz_dr : Inport  Port=3
  Fz_dr1 : Inport  Port=4
  Clock : Clock
  Constant3 : Constant  Value=120
  Constant4 : Constant  Value=0
  Constant5 : Constant  Value=0
  Demux : Demux  Outputs=3
  Demux1 : Demux  Outputs=[57,3,40]
  Gain1 : Gain  Gain=-1  ParamDataTypeStr=double  OutDataTypeStr=double
  Integrator : Integrator
  MATLAB Function : MATLAB Function  TreatAsAtomicUnit=on
  Mux : Mux  Inputs=7
  S-Function : S-Function  FunctionName=hose3D_n_air_Fv_correction  SFunctionDeploymentMode=off  EnableBusSupport=off
  Scope{,1..4,6} (6 alike) : Scope
  Sum : Sum  Inputs=|++
  To Workspace : ToWorkspace  VariableName=output_3D  SampleTime=-1
  To Workspace1 : ToWorkspace  VariableName=output_dr1  SampleTime=-1
  To Workspace3 : ToWorkspace  VariableName=input_x  SampleTime=-1
  To Workspace4 : ToWorkspace  VariableName=input_y  SampleTime=-1
  To Workspace5 : ToWorkspace  VariableName=input_z  SampleTime=-1
  Pxdr_tk : Outport
  Pydr_tk : Outport  Port=2
  Pzdr_tk : Outport  Port=3
  output_3D : Outport  Port=4
  Pos_dr2tx : Outport  Port=5
  wires:
  Mux/1 -> S-Function/1
  Constant3/1 -> Mux/4
  Constant4/1 -> Mux/5
  Constant5/1 -> Mux/6
  Fy_dr/1 -> Mux/2, To Workspace4/1
  Fz_dr/1 -> Scope2/1, Gain1/1
  Fx_dr/1 -> To Workspace3/1, Mux/1
  Demux1/1 -> Scope1/1
  Demux1/3 -> Scope6/1
  Demux1/2 -> Pos_dr2tx/1, Demux/1, To Workspace1/1, Scope3/1
  Demux/1 -> Pxdr_tk/1
  Demux/2 -> Pydr_tk/1
  Demux/3 -> Pzdr_tk/1
  Gain1/1 -> Mux/3, To Workspace5/1
  S-Function/1 -> Demux1/1, Scope/1, output_3D/1, To Workspace/1
  Fz_dr1/1 -> Integrator/1
  Sum/1 -> Scope4/1, Mux/7
  Integrator/1 -> Sum/1
  Clock/1 -> MATLAB Function/1(u)
  MATLAB Function/1(y) -> Sum/2

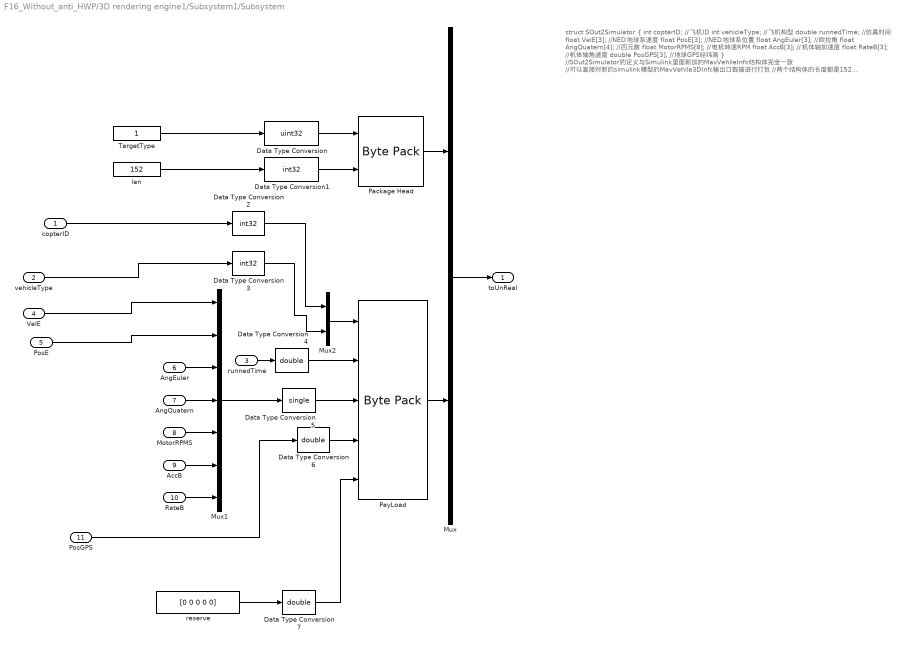
== system F16_Without_anti_HWP/3D rendering engine1/Subsystem1/Subsystem ==
  note: struct SOut2Simulator
      | {
      | int copterID; //飞机ID
      | int vehicleType; //飞机构型
      | double runnedTime; //仿真时间
      | float VelE[3]; //NED地球系速度
      | float PosE[3]; //NED地球系位置
      | float AngEuler[3]; //欧拉角
      | float AngQuatern[4]; //四元数
      | float MotorRPMS[8]; //电机转速RPM
      | float AccB[3]; //机体轴加速度
      | float RateB[3]; //机体轴角速度
      | double PosGPS[3]; //地球GPS经纬高
      | }
      |
      | //SOut2Simulator的定义与Simulink里面新加的MavVehileInfo结构体完全一致
      | //可以直接对新的simulink模型的MavVehile3DInfo输出口数据进行打包
      | //两个结构体的长度都是152
      | sizeof(SOut2Simulator) = sizeof(MavVehileInfo) = 152
      |
      | 打包封装的结构体为
      | typedef struct _netDataShort
      | {
      | TargetType tg; //这里目前随便填，写1即可 uint32
      | int len; //这个长度为传输结构体长度，目前是152
      | char payload[192]; //这里面前152位存放了SOut2Simulator结构体数据，后面的40位保留
      | }netDataShort;
      |
      | //UDP包的总长度为200
      | sizeof(netDataShort) = 200
      |
      | //发送的UDP端口号为：20010
  copterID : Inport  PortDimensions=1
  vehicleType : Inport  Port=2  PortDimensions=1
  runnedTime : Inport  Port=3  PortDimensions=1
  "VelE " : Inport  Port=4  PortDimensions=3
  PosE : Inport  Port=5  PortDimensions=3
  AngEuler : Inport  Port=6  PortDimensions=3
  AngQuatern : Inport  Port=7  PortDimensions=4
  MotorRPMS : Inport  Port=8  PortDimensions=8
  AccB : Inport  Port=9  PortDimensions=3
  RateB : Inport  Port=10  PortDimensions=3
  PosGPS : Inport  Port=11  PortDimensions=3
  Data Type Conversion : DataTypeConversion  OutDataTypeStr=uint32  SaturateOnIntegerOverflow=off  RndMeth=Floor
  Data Type Conversion1 : DataTypeConversion  OutDataTypeStr=int32  SaturateOnIntegerOverflow=off  RndMeth=Floor
  Data Type Conversion2 : DataTypeConversion  OutDataTypeStr=int32  SaturateOnIntegerOverflow=off  RndMeth=Floor
  Data Type Conversion3 : DataTypeConversion  OutDataTypeStr=int32  SaturateOnIntegerOverflow=off  RndMeth=Floor
  Data Type Conversion4 : DataTypeConversion  OutDataTypeStr=double  SaturateOnIntegerOverflow=off  RndMeth=Floor
  Data Type Conversion5 : DataTypeConversion  OutDataTypeStr=single  SaturateOnIntegerOverflow=off  RndMeth=Floor
  Data Type Conversion6 : DataTypeConversion  OutDataTypeStr=double  SaturateOnIntegerOverflow=off  RndMeth=Floor
  Data Type Conversion7 : DataTypeConversion  OutDataTypeStr=double  SaturateOnIntegerOverflow=off  RndMeth=Floor
  Mux : Mux  Inputs=2
  Mux1 : Mux  Inputs=7
  Mux2 : Mux  Inputs=2
  Package Head : etargetslib/Byte Pack  datatypes={'uint32','int32'}  byteAlign=4
  PayLoad : etargetslib/Byte Pack  datatypes={'int32','double','single','double','double'}  byteAlign=8
  TargetType : Constant  OutDataTypeStr=Inherit: Inherit via back propagation
  len : Constant  Value=152  OutDataTypeStr=Inherit: Inherit via back propagation
  reserve : Constant  Value=[0 0 0 0 0]  OutDataTypeStr=double
  toUnReal : Outport  VectorParamsAs1DForOutWhenUnconnected=off
  wires:
  runnedTime/1 -> Data Type Conversion4/1
  RateB/1 -> Mux1/7
  PayLoad/1 -> Mux/2
  "VelE "/1 -> Mux1/1
  Mux1/1 -> Data Type Conversion5/1
  PosGPS/1 -> Data Type Conversion6/1
  Package Head/1 -> Mux/1
  AccB/1 -> Mux1/6
  Mux/1 -> toUnReal/1
  MotorRPMS/1 -> Mux1/5
  AngQuatern/1 -> Mux1/4
  copterID/1 -> Data Type Conversion2/1
  len/1 -> Data Type Conversion1/1
  vehicleType/1 -> Data Type Conversion3/1
  PosE/1 -> Mux1/2
  TargetType/1 -> Data Type Conversion/1
  reserve/1 -> Data Type Conversion7/1
  Mux2/1 -> PayLoad/1
  AngEuler/1 -> Mux1/3
  Data Type Conversion5/1 -> PayLoad/3
  Data Type Conversion2/1 -> Mux2/1
  Data Type Conversion1/1 -> Package Head/2
  Data Type Conversion6/1 -> PayLoad/4
  Data Type Conversion/1 -> Package Head/1
  Data Type Conversion3/1 -> Mux2/2
  Data Type Conversion4/1 -> PayLoad/2
  Data Type Conversion7/1 -> PayLoad/5

== matlab function F16_Without_anti_HWP/MATLAB Function ==
  data: t input; y output; v input
function y = fcn(t,v)
y=zeros(3,1);
y(1)=-13-10;
y(2)=0.02;
y(3)=5;

if t>10&&t<22
    y(1)=-13-10+(t-10)*11/12;
end

if t>=22 & t<30
    y(1)=-13-10+(22-10)*11/12-(t-22)*1.2;
end

== matlab function F16_Without_anti_HWP/Drague&Tube System/MATLAB Function ==
  data: u input; y output; v input
function y = fcn(u,v)
y=[0;0;0];
if u(1)>0
%     if v(1)>=1
%         y(1)=1000*v(1);
%         if(u(1)>0.05)
%             y(1)= y(1)+10000*u(1);
%         end
%     else
%         if(u(1)>0.05)
%             y(1)=10000*u(1);
%         else
%             y(1)=500*u(1)+100*v(1);
%         end 
%     end
    y(1)=1000*u(1);
    if u(1)>0.01
        y(1)=5000*u(1);
    end
    
    if u(1)>0.02
        y(1)=10000*u(1);
    end  
    %y(1)=y(1)+100*v(1);
    

end


if u(1)>-0.1 && u(2) > 0.05
    y(2)=10000*(u(2)-0.05);
end

if u(1)>-0.1 && u(2) <- 0.05
    y(2)=10000*(u(2)+0.05);
end

if u(1)>-0.1 && u(3) > 0.05
    y(2)=10000*(u(3)-0.05);
end

if u(1)>-0.1 && u(3) <- 0.05
    y(3)=10000*(u(3)+0.05);
end




% if u(1)>-0.15 && u(3) > 0.2
%     if v(3)>=1
%         y(3)=1000*v(3);
%     else
%         y(3)=5000*(u(3)-0.2)+100*v(3);
%     end
% end
% 
% if u(1)>-0.15 && u(3) <- 0.2
%     if v(3)<=-1
%         y(3)=1000*v(3);
%     else
%         y(3)=5000*(u(3)+0.2)+100*v(3);
%     end
% end

== matlab function F16_Without_anti_HWP/SimToVR ==
  data: y output; PosPr1 input; PosTb1 input
function y = SimToVR(PosPr1,PosTb1)
%#codegen

%%函数名：SimToVR
%%用途  ：将软管锥套坐标输出转换为VR输入
%%输入  ：PosPr - 受油机椎管坐标， PlsTb - 软管坐标数据
%%输出  ：VrPos - 软管和受油机VR位置，VrAngle - 旋转角度输出
%%作者  ：戴训华
%%时间  ：2014/3/19

PosPr = PosPr1(1:3);
AttitudeRecei = [PosPr1(4);-PosPr1(6);PosPr1(5)-0.115609];

PosTb = PosTb1(1:60);

VrAngle = zeros(22*4,1);
VrPos = zeros(22*3,1);


for j = 1:21                        %前20为软管坐标数据，后1为软管平滑过渡处理
    if j == 1
        pX = [0, 0, 0]';            %软管起点
        pY = PosTb(3*j-2:3*j);      %软杆终点
    elseif j == 21                  %多加一段杆，做过渡
        pX = PosTb(3*j-5:3*j-3);
        pY = [PosTb(3*j-5)-0.7163*cos(8/180*pi),PosTb(3*j-4),PosTb(3*j-3)+0.7163*sin(8/180*pi)]';
    else
        pX = PosTb(3*j-5:3*j-3);
        pY = PosTb(3*j-2:3*j); 
    end
    
    pZ = (pX + pY)/2;               %中点坐标
    pZ = pZ * 8/3;                  %到VR中比例的缩放

    vAxis = [0,0,-1]';               %水平轴
    vTb = pY - pX;                  %杆的方向
    
    axis1 = null([vAxis';vTb']);%获取垂直向量
    vRot = axis1(:,1)';             %得到旋转轴
    
    if vRot(2) < 0
        vRot = -vRot;
    end
    
    VrAngle(4*j-3:4*j-1) = [vRot(1),vRot(3),vRot(2)]';
    VrAngle(4*j) = acos(vAxis'*vTb / sqrt(vAxis'*vAxis * vTb'*vTb));
    
    VrPos(3*j-2:3*j) = [pZ(1),-pZ(3),pZ(2)]';
end
%y = u;
VrAngle(85:88)=[AttitudeRecei(1);AttitudeRecei(2);AttitudeRecei(3);norm(AttitudeRecei)];
pZ = PosPr+[0 -0.1 -0.05]';
pZ = pZ * 8/3;
VrPos(3*22-2:3*22) = [pZ(1),-pZ(3),pZ(2)]';

VrPos(3*21-2) = VrPos(3*21-2)+0.8;
VrPos(3*21-1) = VrPos(3*21-1)+0.1;

y = [VrAngle;VrPos];

== matlab function F16_Without_anti_HWP/Drague&Tube System/Subsystem/MATLAB Function ==
  data: u input; y output
function y = fcn(u)
if u<=8
    y=11-(u*11/8);
    
else
    y=0;
end

== matlab function F16_Without_anti_HWP/SimToUE1 ==
  data: y output; PosRc input; PosTb1 input
function y = SimToVR(PosRc,PosTb1)
%#codegen

%%函数名：SimToVR
%%用途  ：将软管锥套坐标输出转换为VR输入
%%输入  ：PosPr - 受油机坐标， PlsTb - 软管坐标数据
%%输出  ：VrPos - 软管和受油机VR位置，VrAngle - 旋转角度输出
%%作者  ：戴训华
%%时间  ：2014/3/19

PosRc(1) = PosRc(1) - 8.9;
PosRc(2) = PosRc(2) - 0.4;
PosRc(3) = PosRc(3) + 4.5;

Pos_rc2tx = PosRc(1:3);
% add PosPr1(4:6)存储的是受油机的姿态  模型中在输出姿态[phi, theta, psai]后加上了trim_state1=[0;0.1156,0],这里又给减掉了
% 无人机先绕机体系 z 轴旋转 ψ \psiψ，再绕机体系 y 轴旋转 θ \thetaθ，最后绕机体系 x 轴旋转 ϕ \phiϕ，[yaw,pitch,roll]
% AttitudeRecei = [PosPr1(4);-PosPr1(6);PosPr1(5)-0.115609];
AttitudeRecei = [0;0.1156;0];
PosTb = PosTb1(1:60);

% 这里是20根软管+1个锥套+1个受油机 
VrAngle = zeros(22*3,1);
VrPos = zeros(22*3,1);

% 对于发送模型的视觉修正  全部在这里
% 由于这里只管发送 所以必须让前面模型在计算时也考虑这些修正，这样才能把各种计算都对上
hose_delta_pos = [0;0;0];                      % 视觉对齐 让软管都上升1m
drogue_delta_pos =[0;0;.04];                   % 调整锥套的位置 让它和最后一根软管对上 和软管一样先调整1m，再微调 其实就是 hose_delta_pos + [0.85;0;-0.15]
drogue_delta_angle = [0;0;0];                  % 调整锥套的角度 让它和最后一根软管的角度切合 rpy，pitch向上是正向下是负 [0;-8/180*pi;pi]
drogue_visual_pos = [-0.05;0;1.1];             % 这里要将锥套的位置反馈给前面做计算，要将锥套的视觉位置dr2tx+drogue_visual_pos=实际的锥套位置  
                                               % 方法是通过视觉识别得到的dr2cam(z)+cam2rc(z)+dr2tx(z)=rc2tx(z).这里dr2cam是准确的，只有dr2tx可变，所以修正到这里

% add
scale = 1;
for j = 1:21                        %前20为软管坐标数据，后1为软管平滑过渡处理
    if j == 1
        pX = [0, 0, 0]';            %软管起点
        pY = PosTb(3*j-2:3*j);      %软杆终点
                                    % 不用平滑的 直接用锥套的真实位置
    elseif j == 21                  %多加一段杆，做过渡
        pX = PosTb(3*j-5:3*j-3);
        pY = [PosTb(3*j-5)-0.7163*cos(8/180*pi),PosTb(3*j-4),PosTb(3*j-3)+0.7163*sin(8/180*pi)]';
    else
        pX = PosTb(3*j-5:3*j-3);
        pY = PosTb(3*j-2:3*j); 
    end
    
    pZ = (pX + pY)/2;                   %中点坐标

    %到VR中比例的缩放
    pZ = pZ * scale;
    
    vAxis = [0,0,-1]';                  %水平轴
    vTb = pY - pX;                      %杆的方向
    
    axis1 = null([vAxis';vTb']);        %获取垂直向量
    vRot = axis1(:,1)';                 %得到旋转轴
    
    if vRot(2) < 0
        vRot = -vRot;
    end
 
    yaw_xoz = asin(vTb(2) / sqrt(vTb(1)*vTb(1) + vTb(2)*vTb(2)+ vTb(3)*vTb(3)));
    pitch_z = pi - atan(vTb(3) / vTb(1));
%     pitch_z = atan(vTb(3) / vTb(1));
    roll = 0;   % 圆柱形hose，不用计算roll   
    VrAngle(3*j-2:3*j) = [yaw_xoz, pitch_z, roll];
    % 视觉对齐 让软管都上升hose_delta_posm
    VrPos(3*j-2:3*j) = [pZ(1);pZ(2);pZ(3)] + hose_delta_pos;
end
% add 发送的是受油机的位置
VrAngle(64:66)=[AttitudeRecei(1);AttitudeRecei(2);AttitudeRecei(3)];

pZ = Pos_rc2tx;
pZ = pZ * scale;
VrPos(3*22-2:3*22) = [pZ(1),pZ(2),pZ(3)]';


tmp1 = VrPos(1:60,:);                               % 软管位置
tmp2 = VrPos(61:63,:) + drogue_delta_pos;           % 锥套位置
tmp3 = VrPos(64:66,:) ;                             % 受油机位置 
tmp4 = VrAngle(1:60,:);                             % 软管角度
tmp5 = tmp4(58:60) + drogue_delta_angle;            % 锥套角度 使用的是最后一根软管的角度
tmp6 = VrAngle(64:66,:);                            % 受油机角度

tmp=[tmp1;tmp4;tmp2;tmp5;tmp3;tmp6];
y = tmp;

% 发送反馈给前面的锥套位置由于视觉上有差异，所以需要修正 但是实际上发送的是tmp2，并没有发送调整过的值 
Pos_dr2tx=tmp2+drogue_visual_pos;

== matlab function F16_Without_anti_HWP/Drague&Tube System/MATLAB Function1 ==
  data: u input; y output; y1 output; y2 output; y3 output
function [y,y1,y2,y3] = fcn(u)
ll=zeros(20,1);
for i=1:20
    if i==1
       uk_1 = [0;0;0];
    else
        uk_1 = [u(3*(i-1)-2);u(3*(i-1)-2+1);u(3*(i-1)-2+2)];
    end
    uk = [u(3*(i)-2);u(3*(i)-2+1);u(3*(i)-2+2)];
    
    ll(i)=sqrt((uk(1)-uk_1(1))^2+(uk(2)-uk_1(2))^2+(uk(3)-uk_1(3))^2);
end

y = sum(ll);

y1= sqrt((u(58))^2+(u(59))^2+(u(60))^2);
y2 = y1-y;

y3  = 0;

if y2 <-0.1
    y3 = -0.5*y2;
end
